simulink model "Active_Aero_System"  (R2019b)
settings: Solver=VariableStepAuto  StartTime=0.0  StopTime=10.0  RelTol=1e-3
undefined symbols (not defined in the file): Cnst_ExecTime_S, Cnst_Grav, Cnst_Veh_CGx_M, Cnst_Veh_CGz_M, Cnst_Veh_Mass_KG, Cnst_Veh_MaxFrc_N, Cnst_Veh_WhlBase_M
libraries: Aero_Model_Lib x1
settings Model: OrderedModelArguments=off  Creator=creal  LastModifiedBy=creal

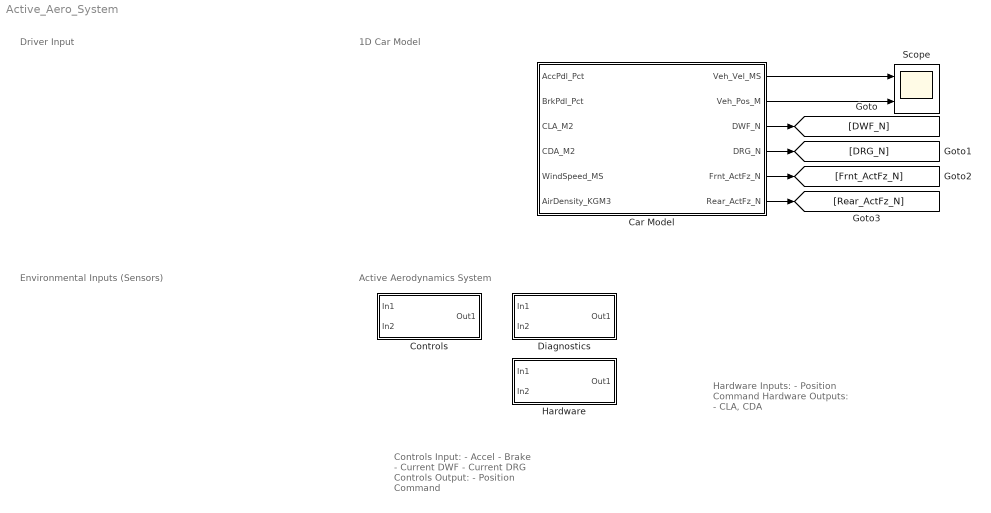
== system Active_Aero_System ==
  note: Hardware Inputs:
      |  - Position Command
      |
      | Hardware Outputs:
      |  - CLA, CDA
  note: Controls Input:
      |  - Accel
      |  - Brake
      |  - Current DWF
      |  - Current DRG
      |
      | Controls Output:
      |  - Position Command
  note: Driver Input
  note: Active Aerodynamics System
  note: 1D Car Model
  note: Environmental Inputs (Sensors)
  Car Model : Subsystem
  Controls : Subsystem
  Diagnostics : Subsystem
  Hardware : Subsystem
  Scope : Scope  NumInputPorts=2
  wires:
  Car Model/1(Veh_Vel_MS) -> Scope/1
  Car Model/2(Veh_Pos_M) -> Scope/2
  Car Model/3(DWF_N) -> [DWF_N]
  Car Model/6(Rear_ActFz_N) -> [Rear_ActFz_N]
  Car Model/5(Frnt_ActFz_N) -> [Frnt_ActFz_N]
  Car Model/4(DRG_N) -> [DRG_N]

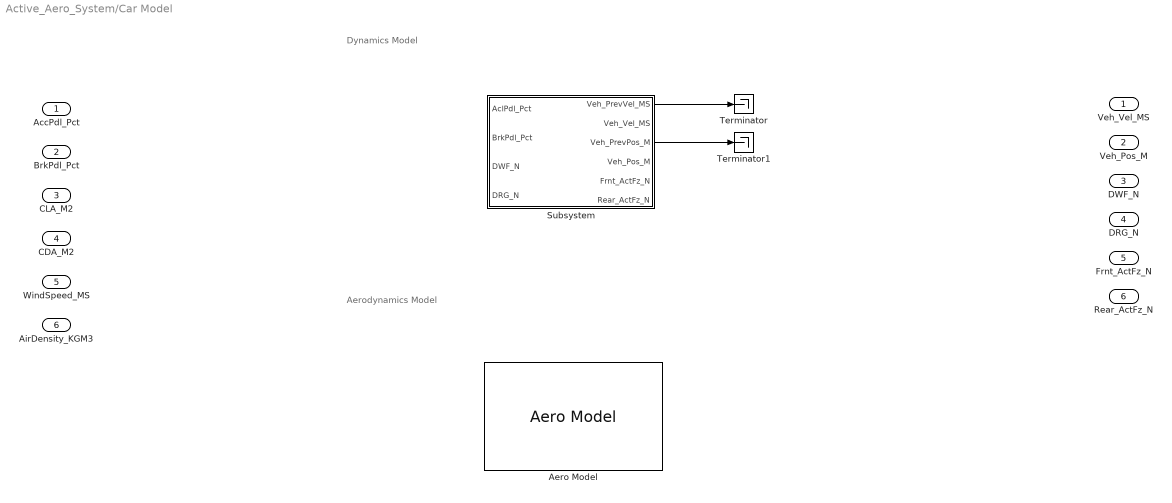
== system Active_Aero_System/Car Model ==
  note: Dynamics Model
  note: Aerodynamics Model
  AccPdl_Pct : Inport
  BrkPdl_Pct : Inport  Port=2
  CLA_M2 : Inport  Port=3
  CDA_M2 : Inport  Port=4
  WindSpeed_MS : Inport  Port=5
  AirDensity_KGM3 : Inport  Port=6
  Aero Model : Aero_Model_Lib/Aero Model  SystemSampleTime=-1  Latency=0  AutoFrameSizeCalculation=off
  Subsystem : Subsystem
  Terminator : Terminator
  Terminator1 : Terminator
  Veh_Vel_MS : Outport
  Veh_Pos_M : Outport  Port=2
  DWF_N : Outport  Port=3
  DRG_N : Outport  Port=4
  Frnt_ActFz_N : Outport  Port=5
  Rear_ActFz_N : Outport  Port=6
  wires:
  Subsystem/1(Veh_PrevVel_MS) -> Terminator/1
  Subsystem/3(Veh_PrevPos_M) -> Terminator1/1

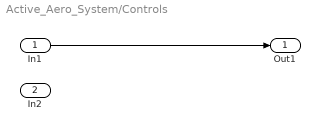
== system Active_Aero_System/Controls ==
  In1 : Inport
  In2 : Inport  Port=2
  Out1 : Outport
  wires:
  In1/1 -> Out1/1

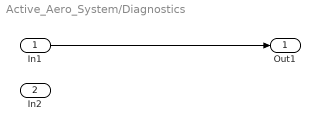
== system Active_Aero_System/Diagnostics ==
  In1 : Inport
  In2 : Inport  Port=2
  Out1 : Outport
  wires:
  In1/1 -> Out1/1

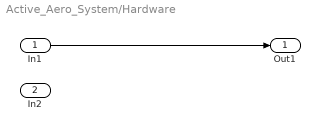
== system Active_Aero_System/Hardware ==
  In1 : Inport
  In2 : Inport  Port=2
  Out1 : Outport
  wires:
  In1/1 -> Out1/1

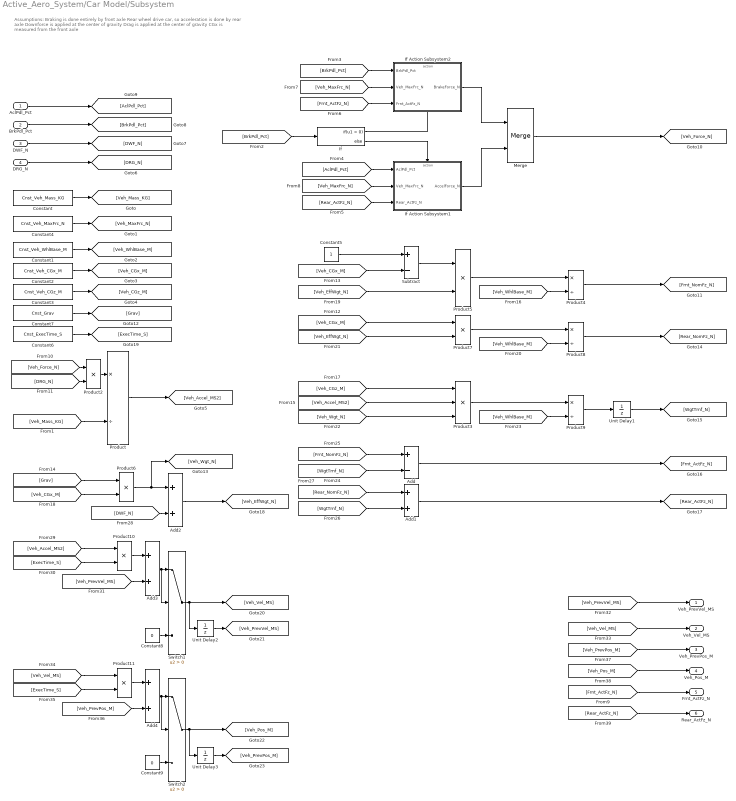
== system Active_Aero_System/Car Model/Subsystem ==
  note: Assumptions:
      | Braking is done entirely by front axle
      | Rear wheel drive car, so acceleration is done by rear axle
      | Downforce is applied at the center of gravity
      | Drag is applied at the center of gravity
      | CGx is measured from the front axle
  "AclPdl_Pct " : Inport
  "BrkPdl_Pct " : Inport  Port=2
  DWF_N : Inport  Port=3
  DRG_N : Inport  Port=4
  Add : Sum  Inputs=+-
  Add{1..4} (4 alike) : Sum
  Constant : Constant  Value=Cnst_Veh_Mass_KG
  Constant1 : Constant  Value=Cnst_Veh_WhlBase_M
  Constant2 : Constant  Value=Cnst_Veh_CGx_M
  Constant3 : Constant  Value=Cnst_Veh_CGz_M
  Constant4 : Constant  Value=Cnst_Veh_MaxFrc_N
  Constant5 : Constant
  Constant6 : Constant  Value=Cnst_ExecTime_S
  Constant7 : Constant  Value=Cnst_Grav
  Constant8 : Constant  Value=0
  Constant9 : Constant  Value=0
  If : If
  If Action Subsystem1 : Subsystem  TreatAsAtomicUnit=on
  If Action Subsystem2 : Subsystem  TreatAsAtomicUnit=on
  Merge : Merge
  Product{,4,8..9} (4 alike) : Product  Inputs=*/
  Product{2,5..7,10..11} (6 alike) : Product
  Product3 : Product  Inputs=3
  Subtract : Sum  Inputs=+-
  Switch1 : Switch  Criteria=u2 > Threshold
  Switch2 : Switch  Criteria=u2 > Threshold
  Unit Delay1 : UnitDelay  SampleTime=-1  HasFrameUpgradeWarning=on
  Unit Delay2 : UnitDelay  SampleTime=-1  HasFrameUpgradeWarning=on
  Unit Delay3 : UnitDelay  SampleTime=-1  HasFrameUpgradeWarning=on
  Veh_PrevVel_MS : Outport
  Veh_Vel_MS : Outport  Port=2
  Veh_PrevPos_M : Outport  Port=3
  Veh_Pos_M : Outport  Port=4
  Frnt_ActFz_N : Outport  Port=5
  Rear_ActFz_N : Outport  Port=6
  wires:
  Constant/1 -> [Veh_Mass_KG]
  Constant3/1 -> [Veh_CGz_M]
  Constant2/1 -> [Veh_CGx_M]
  Constant1/1 -> [Veh_WhlBase_M]
  Constant4/1 -> [Veh_MaxFrc_N]
  [Veh_Mass_KG] -> Product/2
  Product/1 -> [Veh_Accel_MS2]
  "AclPdl_Pct "/1 -> [AclPdl_Pct]
  "BrkPdl_Pct "/1 -> [BrkPdl_Pct]
  DWF_N/1 -> [DWF_N]
  DRG_N/1 -> [DRG_N]
  [BrkPdl_Pct] -> If/1
  If/1 -> If Action Subsystem2/Action
  [BrkPdl_Pct] -> If Action Subsystem2/1(BrkPdl_Pct)
  If/2 -> If Action Subsystem1/Action
  If Action Subsystem1/1(AccelForce_N) -> Merge/2
  [Frnt_ActFz_N] -> If Action Subsystem2/3(Frnt_ActFz_N)
  If Action Subsystem2/1(BrakeForce_N) -> Merge/1
  Merge/1 -> [Veh_Force_N]
  Product2/1 -> Product/1
  [Veh_Force_N] -> Product2/1
  [DRG_N] -> Product2/2
  Constant5/1 -> Subtract/1
  [Veh_CGx_M] -> Subtract/2
  [Veh_Accel_MS2] -> Product3/2
  [Veh_CGx_M] -> Product7/1
  Subtract/1 -> Product5/1
  Product5/1 -> Product4/1
  [Veh_WhlBase_M] -> Product4/2
  Product4/1 -> [Frnt_NomFz_N]
  [Veh_CGz_M] -> Product3/1
  Constant7/1 -> [Grav]
  [Veh_CGx_M] -> Product6/2
  Product6/1 -> Add2/1, [Veh_Wgt_N]
  [Grav] -> Product6/1
  [Veh_EffWgt_N] -> Product5/2
  Product7/1 -> Product8/1
  [Veh_WhlBase_M] -> Product8/2
  [Veh_EffWgt_N] -> Product7/2
  [Veh_Wgt_N] -> Product3/3
  Product3/1 -> Product9/1
  [Veh_WhlBase_M] -> Product9/2
  Product9/1 -> Unit Delay1/1
  Add/1 -> [Frnt_ActFz_N]
  Add1/1 -> [Rear_ActFz_N]
  Product8/1 -> [Rear_NomFz_N]
  [DWF_N] -> Add2/2
  Add2/1 -> [Veh_EffWgt_N]
  Constant6/1 -> [ExecTime_S]
  [Veh_Accel_MS2] -> Product10/1
  [ExecTime_S] -> Product10/2
  Product10/1 -> Add3/1
  [Veh_PrevVel_MS] -> Add3/2
  Unit Delay2/1 -> [Veh_PrevVel_MS]
  Add3/1 -> Switch1/2, Switch1/1
  Switch1/1 -> [Veh_Vel_MS], Unit Delay2/1
  Constant8/1 -> Switch1/3
  [Veh_PrevVel_MS] -> Veh_PrevVel_MS/1
  [Veh_Vel_MS] -> Veh_Vel_MS/1
  Unit Delay1/1 -> [WgtTrnf_N]
  [AclPdl_Pct] -> If Action Subsystem1/1(AclPdl_Pct)
  [Rear_ActFz_N] -> If Action Subsystem1/3(Rear_ActFz_N)
  Constant9/1 -> Switch2/3
  Switch2/1 -> Unit Delay3/1, [Veh_Pos_M]
  Add4/1 -> Switch2/1, Switch2/2
  Unit Delay3/1 -> [Veh_PrevPos_M]
  [Veh_PrevPos_M] -> Add4/2
  Product11/1 -> Add4/1
  [ExecTime_S] -> Product11/2
  [Veh_Vel_MS] -> Product11/1
  [Veh_Pos_M] -> Veh_Pos_M/1
  [Veh_PrevPos_M] -> Veh_PrevPos_M/1
  [WgtTrnf_N] -> Add/2
  [Frnt_NomFz_N] -> Add/1
  [WgtTrnf_N] -> Add1/2
  [Rear_NomFz_N] -> Add1/1
  [Veh_MaxFrc_N] -> If Action Subsystem2/2(Veh_MaxFrc_N)
  [Veh_MaxFrc_N] -> If Action Subsystem1/2(Veh_MaxFrc_N)
  [Frnt_ActFz_N] -> Frnt_ActFz_N/1
  [Rear_ActFz_N] -> Rear_ActFz_N/1

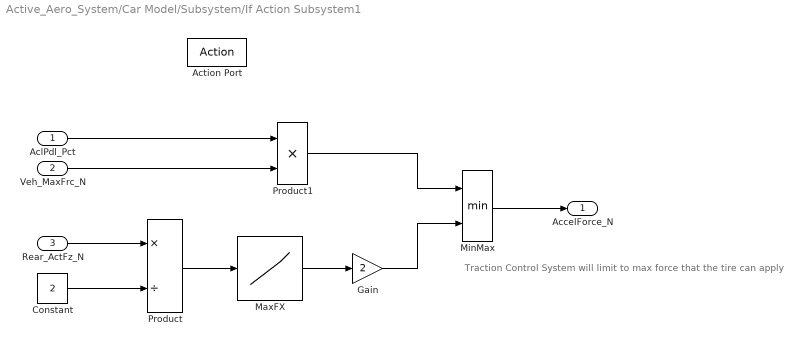
== system Active_Aero_System/Car Model/Subsystem/If Action Subsystem1 ==
  note: Traction Control System will limit to max force that the tire can apply
  AclPdl_Pct : Inport
  Veh_MaxFrc_N : Inport  Port=2
  Rear_ActFz_N : Inport  Port=3
  Action Port : ActionPort  ActionPortLabel=else
  Constant : Constant  Value=2
  Gain : Gain  Gain=2
  "MaxFX " : Lookup_n-D  NumberOfTableDimensions=1  BreakpointsForDimension1=|  Table=|  ExtrapMethod=Clip  InternalRulePriority=Speed  RndMeth=Simplest  InputSameDT=on
      BreakpointsForDimension1=|
      | [333.6
      | 340.34
      | 347.08
      | 353.82
      | 360.56
      | 367.3
      | 374.04
      | 380.78
      | 387.52
      | 394.25
      | 400.99
      | 407.73
      | 414.47
      | 421.21
      | 427.95
      | 434.69
      | 441.43
      | 448.17
      | 454.91
      | 461.65
      | 468.39
      | 475.13
      | 481.87
      | 488.61
      | 495.35
      | 502.08
      | 508.82
      | 515.56
      | 522.3
      | 529.04
      | 535.78
      | 542.52
      | 549.26
      | 556
      | 562.74
      | 569.48
      | 576.22
      | 582.96
      | 589.7
      | 596.44
      | 603.18
      | 609.92
      | 616.65
      | 623.39
      | 630.13
      | 636.87
      | 643.61
      | 650.35
      | 657.09
      | 663.83
      | 670.57
      | 677.31
      | 684.05
      | 690.79
      | 697.53
      | 704.27
      | 711.01
      | 717.75
      | 724.48
      | 731.22
      | 737.96
      | 744.7
      | 751.44
      | 758.18
      | 764.92
      | 771.66
      | 778.4
      | 785.14
      | 791.88
      | 798.62
      | 805.36
      | 812.1
      | 818.84
      | 825.58
      | 832.32
      | 839.05
      | 845.79
      | 852.53
      | 859.27
      | 866.01
      | 872.75
      | 879.49
      | 886.23
      | 892.97
      | 899.71
      | 906.45
      | 913.19
      | 919.93
      | 926.67
      | 933.41
      | 940.15
      | 946.88
      | 953.62
      | 960.36
      | 967.1
      | 973.84
      | 980.58
      | 987.32
      | 994.06
      | 1000.8]
      Table=|
      | [870.52
      | 884.5
      | 898.49
      | 912.73
      | 926.94
      | 941.16
      | 955.39
      | 969.63
      | 983.88
      | 998.15
      | 1012.4
      | 1026.7
      | 1041.2
      | 1055.7
      | 1070.2
      | 1084.7
      | 1099.2
      | 1113.7
      | 1128.3
      | 1142.9
      | 1157.5
      | 1172.3
      | 1187
      | 1201.8
      | 1216.6
      | 1231.4
      | 1246.1
      | 1261
      | 1276
      | 1291
      | 1306
      | 1321
      | 1336
      | 1351.1
      | 1364.8
      | 1378.5
      | 1392.3
      | 1406
      | 1419.8
      | 1433.6
      | 1447.4
      | 1461.2
      | 1475
      | 1488.9
      | 1502.7
      | 1516.6
      | 1530.5
      | 1544.3
      | 1558.2
      | 1572.1
      | 1586.1
      | 1600
      | 1613.9
      | 1627.9
      | 1641.9
      | 1655.8
      | 1669.8
      | 1683.8
      | 1697.9
      | 1711.9
      | 1726
      | 1740
      | 1754.1
      | 1768.2
      | 1782.4
      | 1796.5
      | 1810.6
      | 1824.3
      | 1838
      | 1851.6
      | 1865.3
      | 1879.1
      | 1892.8
      | 1906.6
      | 1920.4
      | 1934.2
      | 1948
      | 1961.8
      | 1975.6
      | 1989.5
      | 2003.3
      | 2017.2
      | 2031.1
      | 2045
      | 2058.9
      | 2072.8
      | 2086.7
      | 2100.7
      | 2114.6
      | 2128.6
      | 2142.6
      | 2156.6
      | 2170.6
      | 2184.6
      | 2198.6
      | 2212.6
      | 2226.7
      | 2240.8
      | 2254.8
      | 2268.9]
  MinMax : MinMax  Inputs=2
  Product : Product  Inputs=*/
  Product1 : Product
  AccelForce_N : Outport
  wires:
  Rear_ActFz_N/1 -> Product/1
  AclPdl_Pct/1 -> Product1/1
  Constant/1 -> Product/2
  Product/1 -> "MaxFX "/1
  Veh_MaxFrc_N/1 -> Product1/2
  MinMax/1 -> AccelForce_N/1
  "MaxFX "/1 -> Gain/1
  Gain/1 -> MinMax/2
  Product1/1 -> MinMax/1

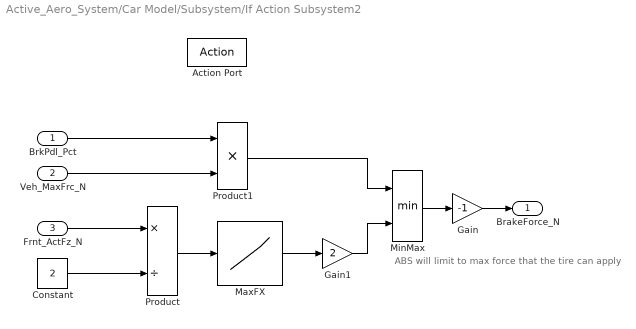
== system Active_Aero_System/Car Model/Subsystem/If Action Subsystem2 ==
  note: ABS will limit to max force that the tire can apply
  BrkPdl_Pct : Inport
  Veh_MaxFrc_N : Inport  Port=2
  Frnt_ActFz_N : Inport  Port=3
  Action Port : ActionPort  ActionPortLabel=if(u1 > 0)
  Constant : Constant  Value=2
  Gain : Gain  Gain=-1
  Gain1 : Gain  Gain=2
  "MaxFX " : Lookup_n-D  NumberOfTableDimensions=1  BreakpointsForDimension1=|  Table=|  ExtrapMethod=Clip  InternalRulePriority=Speed  RndMeth=Simplest  InputSameDT=on
      BreakpointsForDimension1=|
      | [333.6
      | 340.34
      | 347.08
      | 353.82
      | 360.56
      | 367.3
      | 374.04
      | 380.78
      | 387.52
      | 394.25
      | 400.99
      | 407.73
      | 414.47
      | 421.21
      | 427.95
      | 434.69
      | 441.43
      | 448.17
      | 454.91
      | 461.65
      | 468.39
      | 475.13
      | 481.87
      | 488.61
      | 495.35
      | 502.08
      | 508.82
      | 515.56
      | 522.3
      | 529.04
      | 535.78
      | 542.52
      | 549.26
      | 556
      | 562.74
      | 569.48
      | 576.22
      | 582.96
      | 589.7
      | 596.44
      | 603.18
      | 609.92
      | 616.65
      | 623.39
      | 630.13
      | 636.87
      | 643.61
      | 650.35
      | 657.09
      | 663.83
      | 670.57
      | 677.31
      | 684.05
      | 690.79
      | 697.53
      | 704.27
      | 711.01
      | 717.75
      | 724.48
      | 731.22
      | 737.96
      | 744.7
      | 751.44
      | 758.18
      | 764.92
      | 771.66
      | 778.4
      | 785.14
      | 791.88
      | 798.62
      | 805.36
      | 812.1
      | 818.84
      | 825.58
      | 832.32
      | 839.05
      | 845.79
      | 852.53
      | 859.27
      | 866.01
      | 872.75
      | 879.49
      | 886.23
      | 892.97
      | 899.71
      | 906.45
      | 913.19
      | 919.93
      | 926.67
      | 933.41
      | 940.15
      | 946.88
      | 953.62
      | 960.36
      | 967.1
      | 973.84
      | 980.58
      | 987.32
      | 994.06
      | 1000.8]
      Table=|
      | [870.52
      | 884.5
      | 898.49
      | 912.73
      | 926.94
      | 941.16
      | 955.39
      | 969.63
      | 983.88
      | 998.15
      | 1012.4
      | 1026.7
      | 1041.2
      | 1055.7
      | 1070.2
      | 1084.7
      | 1099.2
      | 1113.7
      | 1128.3
      | 1142.9
      | 1157.5
      | 1172.3
      | 1187
      | 1201.8
      | 1216.6
      | 1231.4
      | 1246.1
      | 1261
      | 1276
      | 1291
      | 1306
      | 1321
      | 1336
      | 1351.1
      | 1364.8
      | 1378.5
      | 1392.3
      | 1406
      | 1419.8
      | 1433.6
      | 1447.4
      | 1461.2
      | 1475
      | 1488.9
      | 1502.7
      | 1516.6
      | 1530.5
      | 1544.3
      | 1558.2
      | 1572.1
      | 1586.1
      | 1600
      | 1613.9
      | 1627.9
      | 1641.9
      | 1655.8
      | 1669.8
      | 1683.8
      | 1697.9
      | 1711.9
      | 1726
      | 1740
      | 1754.1
      | 1768.2
      | 1782.4
      | 1796.5
      | 1810.6
      | 1824.3
      | 1838
      | 1851.6
      | 1865.3
      | 1879.1
      | 1892.8
      | 1906.6
      | 1920.4
      | 1934.2
      | 1948
      | 1961.8
      | 1975.6
      | 1989.5
      | 2003.3
      | 2017.2
      | 2031.1
      | 2045
      | 2058.9
      | 2072.8
      | 2086.7
      | 2100.7
      | 2114.6
      | 2128.6
      | 2142.6
      | 2156.6
      | 2170.6
      | 2184.6
      | 2198.6
      | 2212.6
      | 2226.7
      | 2240.8
      | 2254.8
      | 2268.9]
  MinMax : MinMax  Inputs=2
  Product : Product  Inputs=*/
  Product1 : Product
  BrakeForce_N : Outport
  wires:
  Frnt_ActFz_N/1 -> Product/1
  BrkPdl_Pct/1 -> Product1/1
  Veh_MaxFrc_N/1 -> Product1/2
  Product1/1 -> MinMax/1
  Product/1 -> "MaxFX "/1
  Constant/1 -> Product/2
  Gain/1 -> BrakeForce_N/1
  MinMax/1 -> Gain/1
  "MaxFX "/1 -> Gain1/1
  Gain1/1 -> MinMax/2
